simulink model "Satellite_Attitude_Controller_Design"  (R2021b)
settings: Solver=VariableStepAuto  StartTime=0.0  StopTime=10.0  RelTol=1e-3
libraries: simulink x1
settings Model: Creator=rocke  LastModifiedBy=rocke

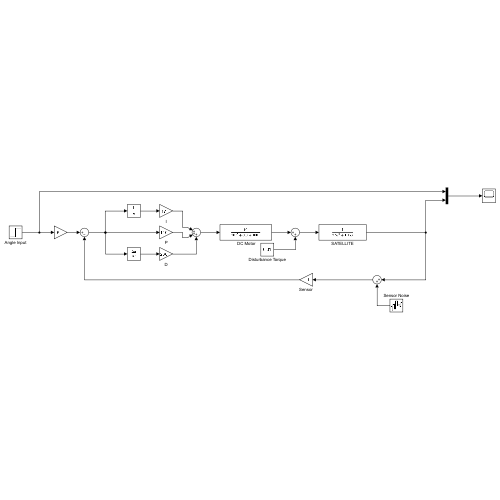
[thumbnail: Simulink's stored preview of the top-level diagram]
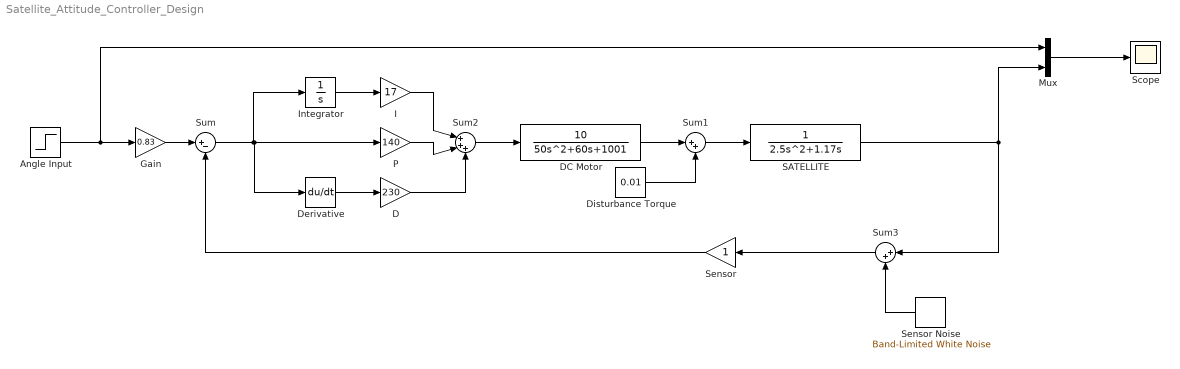
== system Satellite_Attitude_Controller_Design ==
  " DC Motor" : TransferFcn  Numerator=10  Denominator=[50 60 1001]
  Angle Input : Step  After=0.68  SampleTime=0
  D : Gain  Gain=230
  Derivative : Derivative
  Disturbance Torque : Constant  Value=0.01
  Gain : Gain  Gain=0.83
  I : Gain  Gain=17
  Integrator : Integrator
  Mux : Mux  Inputs=2
  P : Gain  Gain=140
  SATELLITE : TransferFcn  Denominator=[2.5 1.17 0]
  Scope : Scope
  Sensor : Gain
  Sensor Noise : simulink/Sources/Band-Limited White Noise  Cov=[0.001]  Ts=0.1  seed=[23341]
  Sum : Sum  Inputs=|+-
  Sum1 : Sum  Inputs=|++
  Sum2 : Sum  Inputs=|+++
  Sum3 : Sum  Inputs=|++
  wires:
  Disturbance Torque/1 -> Sum1/2
  " DC Motor"/1 -> Sum1/1
  Sum1/1 -> SATELLITE/1
  Angle Input/1 -> Gain/1, Mux/1
  Mux/1 -> Scope/1
  Sum/1 -> Integrator/1, Derivative/1, P/1
  Sensor/1 -> Sum/2
  P/1 -> Sum2/2
  Sum2/1 -> " DC Motor"/1
  I/1 -> Sum2/1
  D/1 -> Sum2/3
  Derivative/1 -> D/1
  Integrator/1 -> I/1
  SATELLITE/1 -> Sum3/1, Mux/2
  Gain/1 -> Sum/1
  Sensor Noise/1 -> Sum3/2
  Sum3/1 -> Sensor/1
